simulink model "motor_control"  (R2022b)
settings: Solver=FixedStepAuto  StartTime=0.0  StopTime=10  FixedStep=1e-6  RelTol=1e-3
libraries: spsIGBTDiodeLib x4, spsDCMachineLib x1, spsDCVoltageSourceLib x1, simulink x1, spsSeriesRLCBranchLib x1, spsVoltageMeasurementLib x1, spspowerguiLib x1
settings Model: Creator=91809  LastModifiedBy=91809

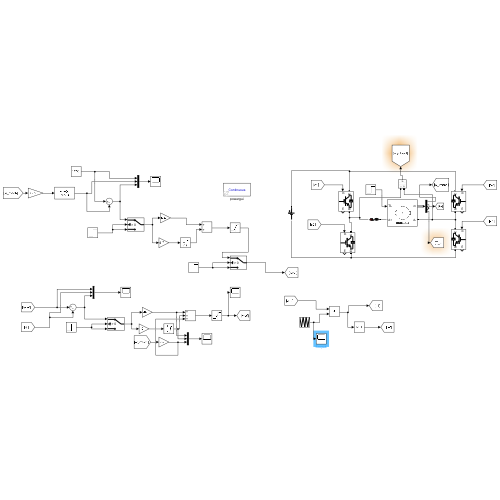
[thumbnail: Simulink's stored preview of the top-level diagram]
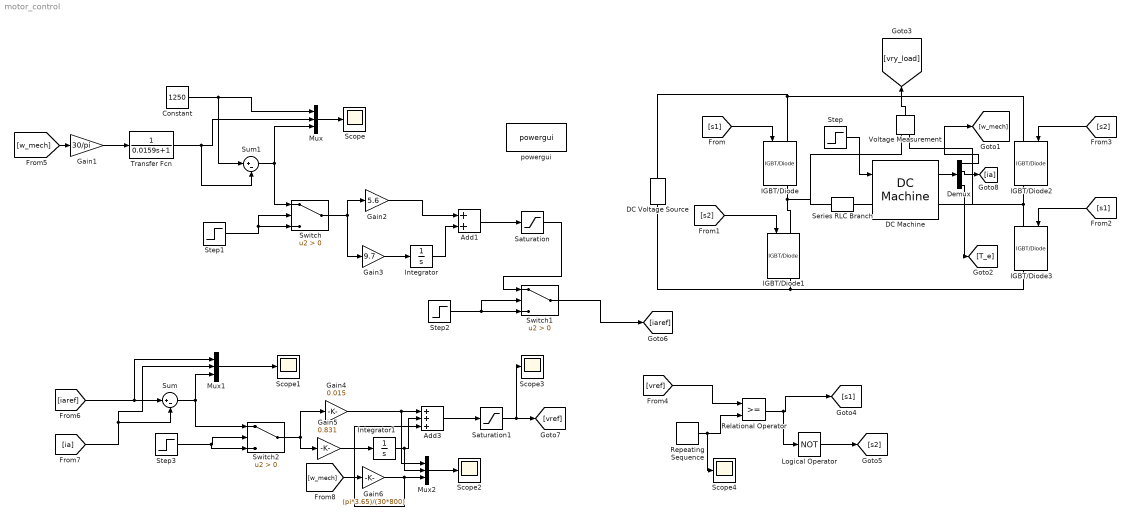
== system motor_control ==
  Add1 : Sum
  Add3 : Sum  Inputs=+++
  Constant : Constant  Value=1250
  DC Machine : spsDCMachineLib/DC Machine  PresetModel=No  MechanicalLoad=Torque TL  FieldType=Permanent magnet  ShowDetailedParameters=on  MeasurementBus=off  RLa="[ 0.052  0.001]"  RLf="[ 240  120]"  Laf=1.8  MachineConstant=Torque constant (N.m/A)  Ke=1.8  Kt=3.65  J=5  Bm=0  Tf=0  w0=0  Ifinit=1  TsPowergui=0  TsBlock=-1
  DC Voltage Source : spsDCVoltageSourceLib/DC Voltage Source  Amplitude=800  Measurements=None
  Demux : Demux
  Gain1 : Gain  Gain=30/pi
  Gain2 : Gain  Gain=5.6
  Gain3 : Gain  Gain=9.7
  Gain4 : Gain  Gain=0.015
  Gain5 : Gain  Gain=0.831
  Gain6 : Gain  Gain=(pi*3.65)/(30*800)
  IGBT/Diode{,1..3} (4 alike) : spsIGBTDiodeLib/IGBT//Diode  Ron=1e-3  Rs=1e5  Cs=inf  Measurements=on
  Integrator : Integrator  LimitOutput=on  UpperSaturationLimit=400  LowerSaturationLimit=-400
  Integrator1 : Integrator  LimitOutput=on  UpperSaturationLimit=1  LowerSaturationLimit=-1
  Logical Operator : Logic  Operator=NOT  AllPortsSameDT=off  OutDataTypeStr=boolean
  Mux : Mux  Inputs=3
  Mux1 : Mux  Inputs=3
  Mux2 : Mux  Inputs=3
  Relational Operator : RelationalOperator  OutDataTypeStr=boolean  RndMeth=Simplest  InputSameDT=off
  Repeating Sequence : simulink/Sources/Repeating Sequence  rep_seq_t=[0 0.00025 0.0005]  rep_seq_y=[1 -1 1]
  Saturation : Saturate  UpperLimit=400  LowerLimit=-400
  Saturation1 : Saturate  UpperLimit=1  LowerLimit=-1
  Scope{,1..4} (5 alike) : Scope
  Series RLC Branch : spsSeriesRLCBranchLib/Series RLC Branch  LConnTagsString=__new0  RConnTagsString=__new0  BranchType=RL  Resistance=0.001  Inductance=9e-3  SetiL0=off  InitialCurrent=0  Capacitance=1e-6  Setx0=off  InitialVoltage=0  Measurements=None
  Step : Step  Time=0.5  After=550  SampleTime=0
  Step1 : Step  Time=0.2  SampleTime=0
  Step2 : Step  Time=0.5  SampleTime=0
  Step3 : Step  Time=0.05  SampleTime=0
  Sum : Sum  Inputs=|+-
  Sum1 : Sum  Inputs=|+-
  Switch : Switch  Criteria=u2 > Threshold  SaturateOnIntegerOverflow=off  InputSameDT=off
  Switch1 : Switch  Criteria=u2 > Threshold  SaturateOnIntegerOverflow=off  InputSameDT=off
  Switch2 : Switch  Criteria=u2 > Threshold  SaturateOnIntegerOverflow=off  InputSameDT=off
  Transfer Fcn : TransferFcn  Denominator=[0.0159 1]
  Voltage Measurement : spsVoltageMeasurementLib/Voltage Measurement  PhasorSimulation=off  OutputType=Complex  PSBequivalent=0
  powergui : spspowerguiLib/powergui  Priority=1  SimulationMode=Continuous  SampleTime=1e-6  frequency=60  Iterations=50  frequencyindice=0  Pbase=100e6  ErrMax=1e-4  UnitsV=kV  UnitsW=MW  buscounter=0  FunctionMessages=off  echomessages=off  EnableUseOfTLC=off  CurrentSourceSwitches=off  DisableSnubberDevices=off  DisableRonSwitches=off  DisableVfSwitches=off  DisplayEquations=off  AutomaticDiscreteSolvers=off  SolverType=Tustin/Backward Euler (TBE)  Interpol=off  ExternalGateDelay=off  methode=off  Ts=100  x0status=blocks  SPID=on  SwTol=0  HookPort=off  NonlinearTolerance=1e-4  nMaxIteration=100  ContinueOnMaxIteration=off  RestoreLinks=warning  ResistiveCurrentMeasurement=off  Frange=[0:2:500]  Ylog=off  Xlog=on  ShowGrid=off  save=off  variable=ZData  structure=0  ZoomFFT=off  StartTime=0.0  cycles=1  DisplayStyle=1  fundamental=60  FreqAxis=off  MaxFrequency=1000  frequencyindicesteady=1  RmsSteady=1  display=off
  wires:
  [s2] -> IGBT/Diode1/1
  [s1] -> IGBT/Diode/1
  Step/1 -> DC Machine/1
  DC Machine/1 -> Demux/1
  Demux/1 -> [w_mech]
  Voltage Measurement/1 -> [vry_load]
  [vref] -> Relational Operator/1
  Relational Operator/1 -> Logical Operator/1, [s1]
  [w_mech] -> Gain1/1
  Gain1/1 -> Transfer Fcn/1
  Constant/1 -> Sum1/1, Mux/1
  Transfer Fcn/1 -> Sum1/2, Mux/2
  Mux/1 -> Scope/1
  Step1/1 -> Switch/3, Switch/2
  Switch/1 -> Gain3/1, Gain2/1
  Gain3/1 -> Integrator/1
  Gain2/1 -> Add1/1
  Integrator/1 -> Add1/2
  Add1/1 -> Saturation/1
  Saturation/1 -> Switch1/1
  Step2/1 -> Switch1/3, Switch1/2
  Mux1/1 -> Scope1/1
  [iaref] -> Mux1/1, Sum/1
  [ia] -> Sum/2, Mux1/2
  Step3/1 -> Switch2/3, Switch2/2
  Switch2/1 -> Gain5/1, Gain4/1
  Gain5/1 -> Integrator1/1
  Gain4/1 -> Mux2/1, Add3/1
  Integrator1/1 -> Mux2/2, Add3/2
  [w_mech] -> Gain6/1
  Gain6/1 -> Add3/3, Mux2/3
  Mux2/1 -> Scope2/1
  Add3/1 -> Saturation1/1
  Saturation1/1 -> Scope3/1, [vref]
  Sum/1 -> Mux1/3, Switch2/1
  Sum1/1 -> Switch/1, Mux/3
  Switch1/1 -> [iaref]
  [s2] -> IGBT/Diode2/1
  [s1] -> IGBT/Diode3/1
  Repeating Sequence/1 -> Scope4/1, Relational Operator/2
  Logical Operator/1 -> [s2]
  Demux/2 -> [ia]
  Demux/4 -> [T_e]
  connections:
  DC Voltage Source/RConn1 -- IGBT/Diode2/LConn1 -- IGBT/Diode/LConn1
  DC Voltage Source/LConn1 -- IGBT/Diode3/RConn1 -- IGBT/Diode1/RConn1
  IGBT/Diode1/LConn1 -- Series RLC Branch/LConn1 -- Voltage Measurement/LConn2 -- IGBT/Diode/RConn1
  IGBT/Diode3/LConn1 -- DC Machine/RConn1 -- Voltage Measurement/LConn1 -- IGBT/Diode2/RConn1
  DC Machine/LConn1 -- Series RLC Branch/RConn1
